simulink model "Problem4"  (R2020b)
settings: Solver=VariableStepAuto  StartTime=0.0  StopTime=10.0  RelTol=1e-3
undefined symbols (not defined in the file): b, J, K, L, R
settings Model: Creator=amolg  LastModifiedBy=amolg

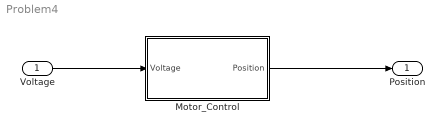
== system Problem4 ==
  Voltage : Inport
  Motor_Control : Subsystem
  Position : Outport
  wires:
  Voltage/1 -> Motor_Control/1(Voltage)
  Motor_Control/1(Position) -> Position/1

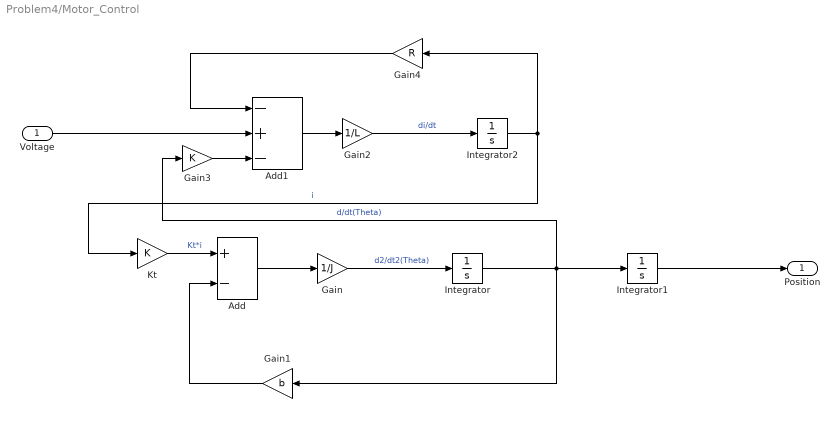
== system Problem4/Motor_Control ==
  Voltage : Inport
  Add : Sum  Inputs=+-
  Add1 : Sum  Inputs=-+-
  Gain : Gain  Gain=1/J
  Gain1 : Gain  Gain=b
  Gain2 : Gain  Gain=1/L
  Gain3 : Gain  Gain=K
  Gain4 : Gain  Gain=R
  Integrator : Integrator
  Integrator1 : Integrator
  Integrator2 : Integrator
  Kt : Gain  Gain=K
  Position : Outport
  wires:
  Gain/1 -> Integrator/1  "d2/dt2(Theta)"
  Integrator/1 -> Gain3/1, Gain1/1, Integrator1/1  "d/dt(Theta)"
  Gain3/1 -> Add1/3
  Voltage/1 -> Add1/2
  Add1/1 -> Gain2/1
  Gain1/1 -> Add/2
  Integrator1/1 -> Position/1
  Add/1 -> Gain/1
  Gain2/1 -> Integrator2/1  "di/dt"
  Kt/1 -> Add/1  "Kt*i"
  Integrator2/1 -> Gain4/1, Kt/1  "i"
  Gain4/1 -> Add1/1
